simulink library "DAQ_lib_HallPositionTorque"  (R2014b)
settings: Solver=ode45  StartTime=0.0  StopTime=10.0  RelTol=1e-3
undefined symbols (not defined in the file): A_lpf_velocity, ANOMALY_INIT, B1_lpf_velocity, B2_lpf_velocity, Calibration, EnableFT, EncoderAngleLimits, EncoderFiltSys, EncoderThreshold, FTCalibration, GearOffsets, IMUAngleLimits, IMUCommand, IMUThreshold, IMUTorsoOffsets, m_XR17D15x, MAX_ANOMALY, MedullaCommand, MicrostrainFiltSys, MODBUS_TIMEOUT, ResetDAQ, ResetYaw, sample_time, standard, STREAMING_TIMEOUT, TareFT, TorsoCOMOffsets, Ts, TsCAN, TsKVH, UseMicrostrainRate
libraries: xpcethercatlib x207, simulink x53, canmsglib x21, speedgoatlib x13, slrtlib x5, speedgoatlib_IO601 x5, dspswit3 x2, dspmtrx3 x2, xpcseriallib x1, SpeedgoatModified x1
(part 6 of 7)

== system DAQ_lib_HallPositionTorque/DAQ Safety Stops IMU Elmo Amplifiers Position and Torque Control with Hall Sensors/DAQ/EtherCATNetwork/EtherCATRobotMicrostrain/LegElmo_1R/Subsystem1/ShutdownControlWord ==
  Action Port : ActionPort
  Constant : Constant  Value=6  OutDataTypeStr=uint16
  ControlWord : Outport
  wires:
  Constant/1 -> ControlWord/1

== system DAQ_lib_HallPositionTorque/DAQ Safety Stops IMU Elmo Amplifiers Position and Torque Control with Hall Sensors/DAQ/EtherCATNetwork/EtherCATRobotMicrostrain/LegElmo_2L/Subsystem1/EnableControlWord ==
  Action Port : ActionPort
  Constant : Constant  Value=15  OutDataTypeStr=uint16
  ControlWord : Outport
  wires:
  Constant/1 -> ControlWord/1

== system DAQ_lib_HallPositionTorque/DAQ Safety Stops IMU Elmo Amplifiers Position and Torque Control with Hall Sensors/DAQ/EtherCATNetwork/EtherCATRobotMicrostrain/LegElmo_2L/Subsystem1/FaultReset ==
  Action Port : ActionPort
  Constant : Constant  Value=128  OutDataTypeStr=uint16
  ControlWord : Outport
  wires:
  Constant/1 -> ControlWord/1

== system DAQ_lib_HallPositionTorque/DAQ Safety Stops IMU Elmo Amplifiers Position and Torque Control with Hall Sensors/DAQ/EtherCATNetwork/EtherCATRobotMicrostrain/LegElmo_2L/Subsystem1/NothingControlWord ==
  Action Port : ActionPort
  Constant : Constant  Value=0  OutDataTypeStr=uint16
  ControlWord : Outport
  wires:
  Constant/1 -> ControlWord/1

== system DAQ_lib_HallPositionTorque/DAQ Safety Stops IMU Elmo Amplifiers Position and Torque Control with Hall Sensors/DAQ/EtherCATNetwork/EtherCATRobotMicrostrain/LegElmo_2L/Subsystem1/ShutdownControlWord ==
  Action Port : ActionPort
  Constant : Constant  Value=6  OutDataTypeStr=uint16
  ControlWord : Outport
  wires:
  Constant/1 -> ControlWord/1

== system DAQ_lib_HallPositionTorque/DAQ Safety Stops IMU Elmo Amplifiers Position and Torque Control with Hall Sensors/DAQ/EtherCATNetwork/EtherCATRobotMicrostrain/LegElmo_2R/Subsystem1/EnableControlWord ==
  Action Port : ActionPort
  Constant : Constant  Value=15  OutDataTypeStr=uint16
  ControlWord : Outport
  wires:
  Constant/1 -> ControlWord/1

== system DAQ_lib_HallPositionTorque/DAQ Safety Stops IMU Elmo Amplifiers Position and Torque Control with Hall Sensors/DAQ/EtherCATNetwork/EtherCATRobotMicrostrain/LegElmo_2R/Subsystem1/FaultReset ==
  Action Port : ActionPort
  Constant : Constant  Value=128  OutDataTypeStr=uint16
  ControlWord : Outport
  wires:
  Constant/1 -> ControlWord/1

== system DAQ_lib_HallPositionTorque/DAQ Safety Stops IMU Elmo Amplifiers Position and Torque Control with Hall Sensors/DAQ/EtherCATNetwork/EtherCATRobotMicrostrain/LegElmo_2R/Subsystem1/NothingControlWord ==
  Action Port : ActionPort
  Constant : Constant  Value=0  OutDataTypeStr=uint16
  ControlWord : Outport
  wires:
  Constant/1 -> ControlWord/1

== system DAQ_lib_HallPositionTorque/DAQ Safety Stops IMU Elmo Amplifiers Position and Torque Control with Hall Sensors/DAQ/EtherCATNetwork/EtherCATRobotMicrostrain/LegElmo_2R/Subsystem1/ShutdownControlWord ==
  Action Port : ActionPort
  Constant : Constant  Value=6  OutDataTypeStr=uint16
  ControlWord : Outport
  wires:
  Constant/1 -> ControlWord/1

== system DAQ_lib_HallPositionTorque/DAQ Safety Stops IMU Elmo Amplifiers Position and Torque Control with Hall Sensors/DAQ/SerialInterfaces/FTCAN/Read_and_Process_Subsystem/CalibrationMatrixBlock/Fx ==
  In : Inport
  Enable : EnablePort
  Out : Outport
  wires:
  In/1 -> Out/1

== system DAQ_lib_HallPositionTorque/DAQ Safety Stops IMU Elmo Amplifiers Position and Torque Control with Hall Sensors/DAQ/SerialInterfaces/FTCAN/Read_and_Process_Subsystem/CalibrationMatrixBlock/Fy ==
  In : Inport
  Enable : EnablePort
  Out : Outport
  wires:
  In/1 -> Out/1

== system DAQ_lib_HallPositionTorque/DAQ Safety Stops IMU Elmo Amplifiers Position and Torque Control with Hall Sensors/DAQ/SerialInterfaces/FTCAN/Read_and_Process_Subsystem/CalibrationMatrixBlock/Fz ==
  In : Inport
  Enable : EnablePort
  Out : Outport
  wires:
  In/1 -> Out/1

== system DAQ_lib_HallPositionTorque/DAQ Safety Stops IMU Elmo Amplifiers Position and Torque Control with Hall Sensors/DAQ/SerialInterfaces/FTCAN/Read_and_Process_Subsystem/CalibrationMatrixBlock/Tx ==
  In : Inport
  Enable : EnablePort
  Out : Outport
  wires:
  In/1 -> Out/1

== system DAQ_lib_HallPositionTorque/DAQ Safety Stops IMU Elmo Amplifiers Position and Torque Control with Hall Sensors/DAQ/SerialInterfaces/FTCAN/Read_and_Process_Subsystem/CalibrationMatrixBlock/Ty ==
  In : Inport
  Enable : EnablePort
  Out : Outport
  wires:
  In/1 -> Out/1

== system DAQ_lib_HallPositionTorque/DAQ Safety Stops IMU Elmo Amplifiers Position and Torque Control with Hall Sensors/DAQ/SerialInterfaces/FTCAN/Read_and_Process_Subsystem/CalibrationMatrixBlock/Tz ==
  In : Inport
  Enable : EnablePort
  Out : Outport
  wires:
  In/1 -> Out/1

== system DAQ_lib_HallPositionTorque/DAQ Safety Stops IMU Elmo Amplifiers Position and Torque Control with Hall Sensors/DAQ/SerialInterfaces/FTCAN/Read_and_Process_Subsystem/CalibrationMatrixBlock1/Fx ==
  In : Inport
  Enable : EnablePort
  Out : Outport
  wires:
  In/1 -> Out/1

== system DAQ_lib_HallPositionTorque/DAQ Safety Stops IMU Elmo Amplifiers Position and Torque Control with Hall Sensors/DAQ/SerialInterfaces/FTCAN/Read_and_Process_Subsystem/CalibrationMatrixBlock1/Fy ==
  In : Inport
  Enable : EnablePort
  Out : Outport
  wires:
  In/1 -> Out/1

== system DAQ_lib_HallPositionTorque/DAQ Safety Stops IMU Elmo Amplifiers Position and Torque Control with Hall Sensors/DAQ/SerialInterfaces/FTCAN/Read_and_Process_Subsystem/CalibrationMatrixBlock1/Fz ==
  In : Inport
  Enable : EnablePort
  Out : Outport
  wires:
  In/1 -> Out/1

== system DAQ_lib_HallPositionTorque/DAQ Safety Stops IMU Elmo Amplifiers Position and Torque Control with Hall Sensors/DAQ/SerialInterfaces/FTCAN/Read_and_Process_Subsystem/CalibrationMatrixBlock1/Tx ==
  In : Inport
  Enable : EnablePort
  Out : Outport
  wires:
  In/1 -> Out/1

== system DAQ_lib_HallPositionTorque/DAQ Safety Stops IMU Elmo Amplifiers Position and Torque Control with Hall Sensors/DAQ/SerialInterfaces/FTCAN/Read_and_Process_Subsystem/CalibrationMatrixBlock1/Ty ==
  In : Inport
  Enable : EnablePort
  Out : Outport
  wires:
  In/1 -> Out/1

== system DAQ_lib_HallPositionTorque/DAQ Safety Stops IMU Elmo Amplifiers Position and Torque Control with Hall Sensors/DAQ/SerialInterfaces/FTCAN/Read_and_Process_Subsystem/CalibrationMatrixBlock1/Tz ==
  In : Inport
  Enable : EnablePort
  Out : Outport
  wires:
  In/1 -> Out/1

== system DAQ_lib_HallPositionTorque/DAQ Safety Stops IMU Elmo Amplifiers Position and Torque Control with Hall Sensors/DAQ/SerialInterfaces/FTCAN/Read_and_Process_Subsystem/ReadCalibrationMatrixRow_FlipFlops/Subsystem ==
  Status : Inport
  Reset : Inport  Port=2
  Enable : EnablePort
  Logical Operator : Logic  IconShape=distinctive  AllPortsSameDT=off  OutDataTypeStr=boolean
  Logical Operator1 : Logic  Operator=NOT  IconShape=distinctive  AllPortsSameDT=off  OutDataTypeStr=boolean
  StatusLatched : Outport
  wires:
  Status/1 -> Logical Operator/1
  Reset/1 -> Logical Operator1/1
  Logical Operator1/1 -> Logical Operator/2
  Logical Operator/1 -> StatusLatched/1

== system DAQ_lib_HallPositionTorque/DAQ Safety Stops IMU Elmo Amplifiers Position and Torque Control with Hall Sensors/DAQ/SerialInterfaces/FTCAN/Read_and_Process_Subsystem/ReadCalibrationMatrixRow_FlipFlops/Subsystem1 ==
  Status : Inport
  Reset : Inport  Port=2
  Enable : EnablePort
  Logical Operator : Logic  IconShape=distinctive  AllPortsSameDT=off  OutDataTypeStr=boolean
  Logical Operator1 : Logic  Operator=NOT  IconShape=distinctive  AllPortsSameDT=off  OutDataTypeStr=boolean
  StatusLatched : Outport
  wires:
  Status/1 -> Logical Operator/1
  Reset/1 -> Logical Operator1/1
  Logical Operator1/1 -> Logical Operator/2
  Logical Operator/1 -> StatusLatched/1

== system DAQ_lib_HallPositionTorque/DAQ Safety Stops IMU Elmo Amplifiers Position and Torque Control with Hall Sensors/DAQ/SerialInterfaces/FTCAN/Read_and_Process_Subsystem/ReadCalibrationMatrixRow_FlipFlops/Subsystem2 ==
  Status : Inport
  Reset : Inport  Port=2
  Enable : EnablePort
  Logical Operator : Logic  IconShape=distinctive  AllPortsSameDT=off  OutDataTypeStr=boolean
  Logical Operator1 : Logic  Operator=NOT  IconShape=distinctive  AllPortsSameDT=off  OutDataTypeStr=boolean
  StatusLatched : Outport
  wires:
  Status/1 -> Logical Operator/1
  Reset/1 -> Logical Operator1/1
  Logical Operator1/1 -> Logical Operator/2
  Logical Operator/1 -> StatusLatched/1

== system DAQ_lib_HallPositionTorque/DAQ Safety Stops IMU Elmo Amplifiers Position and Torque Control with Hall Sensors/DAQ/SerialInterfaces/FTCAN/Read_and_Process_Subsystem/ReadCalibrationMatrixRow_FlipFlops1/Subsystem ==
  Status : Inport
  Reset : Inport  Port=2
  Enable : EnablePort
  Logical Operator : Logic  IconShape=distinctive  AllPortsSameDT=off  OutDataTypeStr=boolean
  Logical Operator1 : Logic  Operator=NOT  IconShape=distinctive  AllPortsSameDT=off  OutDataTypeStr=boolean
  StatusLatched : Outport
  wires:
  Status/1 -> Logical Operator/1
  Reset/1 -> Logical Operator1/1
  Logical Operator1/1 -> Logical Operator/2
  Logical Operator/1 -> StatusLatched/1

== system DAQ_lib_HallPositionTorque/DAQ Safety Stops IMU Elmo Amplifiers Position and Torque Control with Hall Sensors/DAQ/SerialInterfaces/FTCAN/Read_and_Process_Subsystem/ReadCalibrationMatrixRow_FlipFlops1/Subsystem1 ==
  Status : Inport
  Reset : Inport  Port=2
  Enable : EnablePort
  Logical Operator : Logic  IconShape=distinctive  AllPortsSameDT=off  OutDataTypeStr=boolean
  Logical Operator1 : Logic  Operator=NOT  IconShape=distinctive  AllPortsSameDT=off  OutDataTypeStr=boolean
  StatusLatched : Outport
  wires:
  Status/1 -> Logical Operator/1
  Reset/1 -> Logical Operator1/1
  Logical Operator1/1 -> Logical Operator/2
  Logical Operator/1 -> StatusLatched/1

== system DAQ_lib_HallPositionTorque/DAQ Safety Stops IMU Elmo Amplifiers Position and Torque Control with Hall Sensors/DAQ/SerialInterfaces/FTCAN/Read_and_Process_Subsystem/ReadCalibrationMatrixRow_FlipFlops1/Subsystem2 ==
  Status : Inport
  Reset : Inport  Port=2
  Enable : EnablePort
  Logical Operator : Logic  IconShape=distinctive  AllPortsSameDT=off  OutDataTypeStr=boolean
  Logical Operator1 : Logic  Operator=NOT  IconShape=distinctive  AllPortsSameDT=off  OutDataTypeStr=boolean
  StatusLatched : Outport
  wires:
  Status/1 -> Logical Operator/1
  Reset/1 -> Logical Operator1/1
  Logical Operator1/1 -> Logical Operator/2
  Logical Operator/1 -> StatusLatched/1

== system DAQ_lib_HallPositionTorque/DAQ Safety Stops IMU Elmo Amplifiers Position and Torque Control with Hall Sensors/DAQ/SerialInterfaces/FTCAN/Read_and_Process_Subsystem/Select_SetCalibrationMatrixColumn_From_CommandNo/ReadRow1 ==
  Action Port : ActionPort
  Constant : Constant
  OutValue : Outport
  wires:
  Constant/1 -> OutValue/1

== system DAQ_lib_HallPositionTorque/DAQ Safety Stops IMU Elmo Amplifiers Position and Torque Control with Hall Sensors/DAQ/SerialInterfaces/FTCAN/Read_and_Process_Subsystem/Select_SetCalibrationMatrixColumn_From_CommandNo/ReadRow2 ==
  Action Port : ActionPort
  Constant : Constant  Value=2
  OutValue : Outport
  wires:
  Constant/1 -> OutValue/1

== system DAQ_lib_HallPositionTorque/DAQ Safety Stops IMU Elmo Amplifiers Position and Torque Control with Hall Sensors/DAQ/SerialInterfaces/FTCAN/Read_and_Process_Subsystem/Select_SetCalibrationMatrixColumn_From_CommandNo/ReadRow3 ==
  Action Port : ActionPort
  Constant : Constant  Value=3
  OutValue : Outport
  wires:
  Constant/1 -> OutValue/1

== system DAQ_lib_HallPositionTorque/DAQ Safety Stops IMU Elmo Amplifiers Position and Torque Control with Hall Sensors/DAQ/SerialInterfaces/FTCAN/Read_and_Process_Subsystem/Select_SetCalibrationMatrixColumn_From_CommandNo/ReadRow4 ==
  Action Port : ActionPort
  Constant : Constant  Value=4
  OutValue : Outport
  wires:
  Constant/1 -> OutValue/1

== system DAQ_lib_HallPositionTorque/DAQ Safety Stops IMU Elmo Amplifiers Position and Torque Control with Hall Sensors/DAQ/SerialInterfaces/FTCAN/Read_and_Process_Subsystem/Select_SetCalibrationMatrixColumn_From_CommandNo/ReadRow5 ==
  Action Port : ActionPort
  Constant : Constant  Value=5
  OutValue : Outport
  wires:
  Constant/1 -> OutValue/1

== system DAQ_lib_HallPositionTorque/DAQ Safety Stops IMU Elmo Amplifiers Position and Torque Control with Hall Sensors/DAQ/SerialInterfaces/FTCAN/Read_and_Process_Subsystem/Select_SetCalibrationMatrixColumn_From_CommandNo/ReadRow6 ==
  Action Port : ActionPort
  Constant : Constant  Value=6
  OutValue : Outport
  wires:
  Constant/1 -> OutValue/1

== system DAQ_lib_HallPositionTorque/DAQ Safety Stops IMU Elmo Amplifiers Position and Torque Control with Hall Sensors/DAQ/SerialInterfaces/FTCAN/Read_and_Process_Subsystem/Select_SetCalibrationMatrixColumn_From_CommandNo1/ReadRow1 ==
  Action Port : ActionPort
  Constant : Constant
  OutValue : Outport
  wires:
  Constant/1 -> OutValue/1

== system DAQ_lib_HallPositionTorque/DAQ Safety Stops IMU Elmo Amplifiers Position and Torque Control with Hall Sensors/DAQ/SerialInterfaces/FTCAN/Read_and_Process_Subsystem/Select_SetCalibrationMatrixColumn_From_CommandNo1/ReadRow2 ==
  Action Port : ActionPort
  Constant : Constant  Value=2
  OutValue : Outport
  wires:
  Constant/1 -> OutValue/1

== system DAQ_lib_HallPositionTorque/DAQ Safety Stops IMU Elmo Amplifiers Position and Torque Control with Hall Sensors/DAQ/SerialInterfaces/FTCAN/Read_and_Process_Subsystem/Select_SetCalibrationMatrixColumn_From_CommandNo1/ReadRow3 ==
  Action Port : ActionPort
  Constant : Constant  Value=3
  OutValue : Outport
  wires:
  Constant/1 -> OutValue/1

== system DAQ_lib_HallPositionTorque/DAQ Safety Stops IMU Elmo Amplifiers Position and Torque Control with Hall Sensors/DAQ/SerialInterfaces/FTCAN/Read_and_Process_Subsystem/Select_SetCalibrationMatrixColumn_From_CommandNo1/ReadRow4 ==
  Action Port : ActionPort
  Constant : Constant  Value=4
  OutValue : Outport
  wires:
  Constant/1 -> OutValue/1

== system DAQ_lib_HallPositionTorque/DAQ Safety Stops IMU Elmo Amplifiers Position and Torque Control with Hall Sensors/DAQ/SerialInterfaces/FTCAN/Read_and_Process_Subsystem/Select_SetCalibrationMatrixColumn_From_CommandNo1/ReadRow5 ==
  Action Port : ActionPort
  Constant : Constant  Value=5
  OutValue : Outport
  wires:
  Constant/1 -> OutValue/1

== system DAQ_lib_HallPositionTorque/DAQ Safety Stops IMU Elmo Amplifiers Position and Torque Control with Hall Sensors/DAQ/SerialInterfaces/FTCAN/Read_and_Process_Subsystem/Select_SetCalibrationMatrixColumn_From_CommandNo1/ReadRow6 ==
  Action Port : ActionPort
  Constant : Constant  Value=6
  OutValue : Outport
  wires:
  Constant/1 -> OutValue/1

== system DAQ_lib_HallPositionTorque/DAQ Safety Stops IMU Elmo Amplifiers Position and Torque Control with Hall Sensors/DAQ/SerialInterfaces/FTInterface/Subsystem/ComputeCalibratedTorques/Latch ==
  Gauge : Inport
  Tare : EnablePort
  Bias : Outport  InitialOutput=zeros(6,1,'uint16')
  wires:
  Gauge/1 -> Bias/1

== matlab function DAQ_lib_HallPositionTorque/DAQ Safety Stops IMU Elmo Amplifiers Position and Torque Control with Hall Sensors/AdjustForCOMOffset ==
  data: q_in input; q output; TorsoCOMOffsets input
function q = fcn(q_in, TorsoCOMOffsets)
    %#codegen
    
    TorsoCOMRollOffset  = TorsoCOMOffsets(1)*pi/180;
    TorsoCOMPitchOffset = TorsoCOMOffsets(2)*pi/180;
    
    q = q_in;
    q(2)  = q(2)  + TorsoCOMRollOffset;
    q(10) = q(10) - TorsoCOMRollOffset;
    q(13) = q(13) + TorsoCOMRollOffset;
    
    q(3) = q(3) + TorsoCOMPitchOffset;
    q([4:9 11:12]) = q([4:9 11:12]) - TorsoCOMPitchOffset;
end

== matlab function DAQ_lib_HallPositionTorque/DAQ Safety Stops IMU Elmo Amplifiers Position and Torque Control with Hall Sensors/DAQ/EtherCATNetwork/ComputeEulerAngles ==
  data: RkIn input; wk input; RCal input; Reset input; R0In input; ZYX output; dZYX output; Rk output; R0 output; YawRolloverIn input; YawRollover output
function [ZYX, dZYX, Rk, R0, YawRollover] = fcn(RkIn, wk, RCal, Reset, R0In, YawRolloverIn) %#codegen
    % Convert from IMU frame to robot frame and compute Euler angles. The
    % yaw angle is zeroed whenever (Reset) is true.
        
    if (Reset)
        % Compute the rotation matrix which zeroes the initial yaw
        qT0 = M_to_ZYX(RkIn*RCal);
        R0  = Rz(-qT0(1));
    else
        R0 = R0In;
    end
    
    % Transform from IMU to robot frame and zero initial yaw
    Rk = R0*RkIn*RCal;
    
    % Convert Rk to ZYX Euler angles
    ZYX = M_to_ZYX(Rk);
    
    % Unroll yaw
    YawRolloverCount = YawRolloverIn(1);
    PreviousYaw      = YawRolloverIn(2);
    CurrentYaw       = ZYX(1);
    YawRolloverCount = YawRolloverCount + getYawRollover(CurrentYaw, PreviousYaw);
    YawRollover      = [YawRolloverCount; CurrentYaw];
    ZYX(1)           = ZYX(1) + 2*pi*YawRolloverCount;
    
    % Compute Euler angle derivatives
    qzT = ZYX(1);
    qyT = ZYX(2);
    
    if cos(qyT)>1e-3
        dZYX = [0 -sin(qzT) cos(qzT)*cos(qyT); 0 cos(qzT) sin(qzT)*cos(qyT); 1 0 -sin(qyT)]\(R0*RkIn*wk);
    else
        dZYX = [0; 0; 0];
    end
end

function R = Rz(t)
    R = [cos(t) -sin(t) 0; sin(t) cos(t) 0; 0 0 1];
end

function Rollover = getYawRollover(CurrentYaw, PreviousYaw)
    % Determine if a rollover has occurred on yaw angle If a rollover is
    % detected, the output Rollover is either +1 or -1, depending on the
    % direction of the rollover.
  
    if (PreviousYaw>0 && CurrentYaw < (PreviousYaw-pi))
        Rollover = 1;
    elseif (PreviousYaw<0 && CurrentYaw > (PreviousYaw+pi))
        Rollover = -1;
    else
        Rollover = 0;
    end
end

== stateflow chart DAQ_lib_HallPositionTorque/DAQ Safety Stops IMU Elmo Amplifiers Position and Torque Control with Hall Sensors/DAQ/EtherCATNetwork/EncoderFilters/CheckAndFilterEncoder/AnomalyDetection ==
  state Run
    state Nominal
      en, du:
      q_clean = q;
      q_last = q;
      dq_last = dq;
      Counter_last = Counter;
      ErrorCount = 0;
    state MissedPacket
      en, du:
      q_clean = q_last + dq_last*ANOMALY_DT;
      ErrorCount--;
    state Error
      en: dq_last = dq; //dq is delayed to prevent algebraic loops
      en, du:
      ErrorCount++;
      q_clean = q_last + ErrorCount*dq_last*ANOMALY_DT;
    (default) -> Nominal
    Nominal -> MissedPacket [order 1] : [0 && Counter == Counter_last]
    MissedPacket -> Nominal
    Nominal -> Error [order 2] : [check_error()]
    Error -> Nominal [order 2] : [!check_error()]
  state Init
    en, du:
    q_clean = q;
    q_last = q;
    dq_last = dq;
    ErrorCount = 0;
  (default) -> Init
  Init -> Run : [!Reset && after(ANOMALY_INIT, tick)]
  Run -> Init : [Reset]
  Error -> Init [order 1] : [ErrorCount>MAX_ANOMALY]
  data: err function_output boolean; q input size=1; dq input size=1; Counter input; q_clean output double size=1; ErrorCount output double; MAX_ANOMALY parameter double size=1; q_last local double size=1; dq_last local double size=1; ANOMALY_INIT parameter double size=1; q_limits input double size=2; Threshold input size=1; Reset input boolean size=1; ANOMALY_DT input double size=1; Counter_last local double size=1
  function err = check_error:
    | function err = check_error
    |     %#codegen
    |     err = (q<q_limits(1)) || (q>q_limits(2)) ...
    |         || (abs(q - q_clean) > (ErrorCount+1)*Threshold);
    | end

== matlab function DAQ_lib_HallPositionTorque/DAQ Safety Stops IMU Elmo Amplifiers Position and Torque Control with Hall Sensors/DAQ/EtherCATNetwork/EtherCATRobotMicrostrain/ConvertAmpCurrent ==
  data: adc_value input; measuredCurrent output
function measuredCurrent = convert(adc_value)
    %#codegen

    measuredCurrent = (adc_value) * 60.0 / 8192;
end

== matlab function DAQ_lib_HallPositionTorque/DAQ Safety Stops IMU Elmo Amplifiers Position and Torque Control with Hall Sensors/DAQ/EtherCATNetwork/EtherCATRobotMicrostrain/ConvertLogicVoltage ==
  data: adc_value input; logicVoltage output
function logicVoltage = convert(adc_value)
    %#codegen
    
    MEDULLA_ADC_MAX_VOLTS     = 2.70;
    MEDULLA_ADC_OFFSET_COUNTS = 172;
    
    logicVoltage = (adc_value - MEDULLA_ADC_OFFSET_COUNTS) * (MEDULLA_ADC_MAX_VOLTS/(4095.0))  * 6.0;
end

== matlab function DAQ_lib_HallPositionTorque/DAQ Safety Stops IMU Elmo Amplifiers Position and Torque Control with Hall Sensors/DAQ/EtherCATNetwork/EtherCATRobotMicrostrain/ConvertMotorVoltage ==
  data: adc_value input; motorVoltage output
function motorVoltage = convert(adc_value)
    %#codegen
    
    MOTOR_VOLTAGE_C_OFFSET    = 1300.0;
    MOTOR_VOLTAGE_V_CAL       = 60.2;
    MOTOR_VOLTAGE_C_CAL       = 3600.0;
    
    motorVoltage = (adc_value - MOTOR_VOLTAGE_C_OFFSET)*MOTOR_VOLTAGE_V_CAL/(MOTOR_VOLTAGE_C_CAL-MOTOR_VOLTAGE_C_OFFSET);
end

== matlab function DAQ_lib_HallPositionTorque/DAQ Safety Stops IMU Elmo Amplifiers Position and Torque Control with Hall Sensors/DAQ/EtherCATNetwork/EtherCATRobotMicrostrain/ConvertThermistors ==
  data: Temperatures output; adc_value input
function Temperatures  = convert(adc_value)
    %#codegen
    MEDULLA_ADC_MAX_VOLTS     = 2.70;
    MEDULLA_ADC_OFFSET_COUNTS = 172;
    
    processedADCValue = (adc_value - MEDULLA_ADC_OFFSET_COUNTS) * (MEDULLA_ADC_MAX_VOLTS/(4095.0));
    Temperatures = zeros(30,1); % 20141104
    % Temperatures = (1.0./( (1.0/298.15) + (1.0/3988.0)*log(4700.0./((3.26./processedADCValue) - 1.0)/10000))) - 273.15;
end

== matlab function DAQ_lib_HallPositionTorque/DAQ Safety Stops IMU Elmo Amplifiers Position and Torque Control with Hall Sensors/DAQ/EtherCATNetwork/EtherCATRobotMicrostrain/EncodeSwitches ==
  data: Switches input; LimitSwitchesEncoded output
function LimitSwitchesEncoded = EncodeSwitches(Switches)
    LimitSwitchesVec     = uint32(Switches);
    LimitSwitchesEncoded = double(EncodeSwitches(LimitSwitchesVec));
end

== matlab function DAQ_lib_HallPositionTorque/DAQ Safety Stops IMU Elmo Amplifiers Position and Torque Control with Hall Sensors/DAQ/EtherCATNetwork/EtherCATRobotMicrostrain/IMU_Medulla/TypecastAndCast ==
  data: u input uint32; y output
function y = unit32_to_double(u)
    %#codegen
    ys = typecast(u, 'single');
    y  = double(ys);
end

== matlab function DAQ_lib_HallPositionTorque/DAQ Safety Stops IMU Elmo Amplifiers Position and Torque Control with Hall Sensors/DAQ/EtherCATNetwork/EtherCATRobotMicrostrain/IMU_Medulla/TypecastAndCast1 ==
  data: u input uint32; y output
function y = unit32_to_double(u)
    %#codegen
    ys = typecast(u, 'single');
    y  = double(ys);
end

== matlab function DAQ_lib_HallPositionTorque/DAQ Safety Stops IMU Elmo Amplifiers Position and Torque Control with Hall Sensors/DAQ/EtherCATNetwork/EtherCATRobotMicrostrain/IMU_Medulla/TypecastAndCast2 ==
  data: u input uint32; y output
function y = unit32_to_double(u)
    %#codegen
    ys = typecast(u, 'single');
    y  = double(ys);
end

== stateflow chart DAQ_lib_HallPositionTorque/DAQ Safety Stops IMU Elmo Amplifiers Position and Torque Control with Hall Sensors/DAQ/EtherCATNetwork/EtherCATRobotMicrostrain/LegElmo_1L/State Flow ==
  state Start1
    entry:
    ControlWordIndex = 0;
    Enable = 0;
    FaultDetected = 0;
  note: 2 = Medulla Run
  state Initialization
    state SwitchOnDisabled
      entry:
      ControlWordIndex = 1;
      Timeout = 0;
      Enable = 0;
      FaultDetected = 0;
      during:
      Timeout = Timeout + 1;
    state Fault
      entry:
      ControlWordIndex = 3;
      Enable = 0;
      Timeout = 0;
      FaultDetected = 0;
      during:
      Timeout = Timeout + 1;
      ControlWordIndex = 0;
    state ReadyToSwitchOn
      entry:
      ControlWordIndex = 2;
      Timeout = 0;
      Enable = 0;
      FaultDetected = 0;
      during:
      Timeout = Timeout + 1;
    (default) -> SwitchOnDisabled
    SwitchOnDisabled -> Fault [order 2] : [FaultMode == 1]
    Fault -> Fault [order 1] : [Timeout >=20]
    ReadyToSwitchOn -> SwitchOnDisabled [order 2] : [SwitchOnDisabledMode == 1]
    Fault -> SwitchOnDisabled [order 2] : [SwitchOnDisabledMode == 1]
    SwitchOnDisabled -> ReadyToSwitchOn [order 1] : [ReadyToSwitchOnMode == 1]
    ReadyToSwitchOn -> Fault [order 1] : [FaultMode == 1]
  state FaultRunning
    entry:
    ControlWordIndex = 1;
    Enable = 0;
    FaultDetected = 1;
  note: 5 = Error
  note: 4 = Halt
  state Running
    entry:
    FaultDetected = 0;
    ControlWordIndex = 2;
    Enable = 1;
  (default) -> Start1
  Start1 -> Initialization : [MedullaCommand == 2]
  Initialization -> FaultRunning : [MedullaCommand == 4 || MedullaCommand == 5 ]
  Running -> FaultRunning [order 1] : [FaultMode == 1]
  Running -> FaultRunning [order 2] : [MedullaCommand == 4 || MedullaCommand == 5 ]
  ReadyToSwitchOn -> Running [order 3] : [EnabledMode == 1 && FaultMode == 0]
  data: SwitchOnDisabledMode input; EnabledMode input; ReadyToSwitchOnMode input; ControlWordIndex output; Enable output; Timeout local; FaultMode input; FaultDetected output; MedullaCommand input

== stateflow chart DAQ_lib_HallPositionTorque/DAQ Safety Stops IMU Elmo Amplifiers Position and Torque Control with Hall Sensors/DAQ/EtherCATNetwork/EtherCATRobotMicrostrain/LegElmo_1R/State Flow ==
  state Start1
    entry:
    ControlWordIndex = 0;
    Enable = 0;
    FaultDetected = 0;
  note: 2 = Medulla Run
  state Initialization
    state SwitchOnDisabled
      entry:
      ControlWordIndex = 1;
      Timeout = 0;
      Enable = 0;
      FaultDetected = 0;
      during:
      Timeout = Timeout + 1;
    state Fault
      entry:
      ControlWordIndex = 3;
      Enable = 0;
      Timeout = 0;
      FaultDetected = 0;
      during:
      Timeout = Timeout + 1;
      ControlWordIndex = 0;
    state ReadyToSwitchOn
      entry:
      ControlWordIndex = 2;
      Timeout = 0;
      Enable = 0;
      FaultDetected = 0;
      during:
      Timeout = Timeout + 1;
    (default) -> SwitchOnDisabled
    SwitchOnDisabled -> Fault [order 2] : [FaultMode == 1]
    Fault -> Fault [order 1] : [Timeout >=20]
    ReadyToSwitchOn -> SwitchOnDisabled [order 2] : [SwitchOnDisabledMode == 1]
    Fault -> SwitchOnDisabled [order 2] : [SwitchOnDisabledMode == 1]
    SwitchOnDisabled -> ReadyToSwitchOn [order 1] : [ReadyToSwitchOnMode == 1]
    ReadyToSwitchOn -> Fault [order 1] : [FaultMode == 1]
  state FaultRunning
    entry:
    ControlWordIndex = 1;
    Enable = 0;
    FaultDetected = 1;
  note: 5 = Error
  note: 4 = Halt
  state Running
    entry:
    FaultDetected = 0;
    ControlWordIndex = 2;
    Enable = 1;
  (default) -> Start1
  Start1 -> Initialization : [MedullaCommand == 2]
  Initialization -> FaultRunning : [MedullaCommand == 4 || MedullaCommand == 5 ]
  Running -> FaultRunning [order 1] : [FaultMode == 1]
  Running -> FaultRunning [order 2] : [MedullaCommand == 4 || MedullaCommand == 5 ]
  ReadyToSwitchOn -> Running [order 3] : [EnabledMode == 1 && FaultMode == 0]
  data: SwitchOnDisabledMode input; EnabledMode input; ReadyToSwitchOnMode input; ControlWordIndex output; Enable output; Timeout local; FaultMode input; FaultDetected output; MedullaCommand input

== stateflow chart DAQ_lib_HallPositionTorque/DAQ Safety Stops IMU Elmo Amplifiers Position and Torque Control with Hall Sensors/DAQ/EtherCATNetwork/EtherCATRobotMicrostrain/LegElmo_2L/State Flow ==
  state Start1
    entry:
    ControlWordIndex = 0;
    Enable = 0;
    FaultDetected = 0;
  note: 2 = Medulla Run
  state Initialization
    state SwitchOnDisabled
      entry:
      ControlWordIndex = 1;
      Timeout = 0;
      Enable = 0;
      FaultDetected = 0;
      during:
      Timeout = Timeout + 1;
    state Fault
      entry:
      ControlWordIndex = 3;
      Enable = 0;
      Timeout = 0;
      FaultDetected = 0;
      during:
      Timeout = Timeout + 1;
      ControlWordIndex = 0;
    state ReadyToSwitchOn
      entry:
      ControlWordIndex = 2;
      Timeout = 0;
      Enable = 0;
      FaultDetected = 0;
      during:
      Timeout = Timeout + 1;
    (default) -> SwitchOnDisabled
    SwitchOnDisabled -> Fault [order 2] : [FaultMode == 1]
    Fault -> Fault [order 1] : [Timeout >=20]
    ReadyToSwitchOn -> SwitchOnDisabled [order 2] : [SwitchOnDisabledMode == 1]
    Fault -> SwitchOnDisabled [order 2] : [SwitchOnDisabledMode == 1]
    SwitchOnDisabled -> ReadyToSwitchOn [order 1] : [ReadyToSwitchOnMode == 1]
    ReadyToSwitchOn -> Fault [order 1] : [FaultMode == 1]
  state FaultRunning
    entry:
    ControlWordIndex = 1;
    Enable = 0;
    FaultDetected = 1;
  note: 5 = Error
  note: 4 = Halt
  state Running
    entry:
    FaultDetected = 0;
    ControlWordIndex = 2;
    Enable = 1;
  (default) -> Start1
  Start1 -> Initialization : [MedullaCommand == 2]
  Initialization -> FaultRunning : [MedullaCommand == 4 || MedullaCommand == 5 ]
  Running -> FaultRunning [order 1] : [FaultMode == 1]
  Running -> FaultRunning [order 2] : [MedullaCommand == 4 || MedullaCommand == 5 ]
  ReadyToSwitchOn -> Running [order 3] : [EnabledMode == 1 && FaultMode == 0]
  data: SwitchOnDisabledMode input; EnabledMode input; ReadyToSwitchOnMode input; ControlWordIndex output; Enable output; Timeout local; FaultMode input; FaultDetected output; MedullaCommand input

== stateflow chart DAQ_lib_HallPositionTorque/DAQ Safety Stops IMU Elmo Amplifiers Position and Torque Control with Hall Sensors/DAQ/EtherCATNetwork/EtherCATRobotMicrostrain/LegElmo_2R/State Flow ==
  state Start1
    entry:
    ControlWordIndex = 0;
    Enable = 0;
    FaultDetected = 0;
  note: 2 = Medulla Run
  state Initialization
    state SwitchOnDisabled
      entry:
      ControlWordIndex = 1;
      Timeout = 0;
      Enable = 0;
      FaultDetected = 0;
      during:
      Timeout = Timeout + 1;
    state Fault
      entry:
      ControlWordIndex = 3;
      Enable = 0;
      Timeout = 0;
      FaultDetected = 0;
      during:
      Timeout = Timeout + 1;
      ControlWordIndex = 0;
    state ReadyToSwitchOn
      entry:
      ControlWordIndex = 2;
      Timeout = 0;
      Enable = 0;
      FaultDetected = 0;
      during:
      Timeout = Timeout + 1;
    (default) -> SwitchOnDisabled
    SwitchOnDisabled -> Fault [order 2] : [FaultMode == 1]
    Fault -> Fault [order 1] : [Timeout >=20]
    ReadyToSwitchOn -> SwitchOnDisabled [order 2] : [SwitchOnDisabledMode == 1]
    Fault -> SwitchOnDisabled [order 2] : [SwitchOnDisabledMode == 1]
    SwitchOnDisabled -> ReadyToSwitchOn [order 1] : [ReadyToSwitchOnMode == 1]
    ReadyToSwitchOn -> Fault [order 1] : [FaultMode == 1]
  state FaultRunning
    entry:
    ControlWordIndex = 1;
    Enable = 0;
    FaultDetected = 1;
  note: 5 = Error
  note: 4 = Halt
  state Running
    entry:
    FaultDetected = 0;
    ControlWordIndex = 2;
    Enable = 1;
  (default) -> Start1
  Start1 -> Initialization : [MedullaCommand == 2]
  Initialization -> FaultRunning : [MedullaCommand == 4 || MedullaCommand == 5 ]
  Running -> FaultRunning [order 1] : [FaultMode == 1]
  Running -> FaultRunning [order 2] : [MedullaCommand == 4 || MedullaCommand == 5 ]
  ReadyToSwitchOn -> Running [order 3] : [EnabledMode == 1 && FaultMode == 0]
  data: SwitchOnDisabledMode input; EnabledMode input; ReadyToSwitchOnMode input; ControlWordIndex output; Enable output; Timeout local; FaultMode input; FaultDetected output; MedullaCommand input

== stateflow chart DAQ_lib_HallPositionTorque/DAQ Safety Stops IMU Elmo Amplifiers Position and Torque Control with Hall Sensors/DAQ/EtherCATNetwork/IMUFilters/CheckAndFilterIMU/AnomalyDetection ==
  state Run
    state Nominal
      en, du:
      q_clean = q;
      q_last = q;
      dq_last = dq;
      ErrorCount = 0;
    state Error
      en: dq_last = dq; //dq is delayed to prevent algebraic loops
      en, du:
      ErrorCount++;
      q_clean = q_last + ErrorCount*dq_last*ANOMALY_DT;
    (default) -> Nominal
    Nominal -> Error : [check_error()]
    Error -> Nominal [order 2] : [!check_error()]
  state Init
    en, du:
    q_clean = q;
    q_last = q;
    dq_last = dq;
    ErrorCount = 0;
  (default) -> Init
  Init -> Run : [!Reset && after(ANOMALY_INIT, tick)]
  Run -> Init : [Reset]
  Error -> Init [order 1] : [ErrorCount>MAX_ANOMALY]
  data: err function_output boolean; q input size=1; dq input size=1; q_clean output double size=1; ErrorCount output double; MAX_ANOMALY parameter double size=1; q_last local double size=1; dq_last local double size=1; ANOMALY_INIT parameter double size=1; q_limits input double size=2; Threshold input size=1; Reset input boolean size=1; ANOMALY_DT input double size=1
  function err = check_error:
    | function err = check_error
    |     %#codegen
    |     err = (q<q_limits(1)) || (q>q_limits(2)) || (abs(q - q_clean) > (ErrorCount+1)*Threshold); 
    | end

== matlab function DAQ_lib_HallPositionTorque/DAQ Safety Stops IMU Elmo Amplifiers Position and Torque Control with Hall Sensors/DAQ/EtherCATNetwork/ZeroingLegs ==
  data: u input; u_zeroed output
function u_zeroed = ZeroingLegs(u)

% leg_motor_1R_torque_cmd = u(1);
% leg_motor_2R_torque_cmd = u(2);
% hip_motor_3R_torque_cmd = u(3);
% leg_motor_1L_torque_cmd = u(4);
% leg_motor_2L_torque_cmd = u(5);
% hip_motor_3L_torque_cmd = u(6);

u_zeroed = [0;
            0;
            u(3);
            0;
            0;
            u(6)];

end

== matlab function DAQ_lib_HallPositionTorque/DAQ Safety Stops IMU Elmo Amplifiers Position and Torque Control with Hall Sensors/DAQ/EtherCATNetwork/calibrate ==
  data: Calibration input; AbsEncoders input; IncEncoders input; IncEncodersPrev input; AbsAngle output; Reset input; IncAngle output; RolloverIn input; Rollover output; IncCalTickIn input; IncCalTick output
function [AbsAngle, IncAngle, Rollover, IncCalTick] = calibrate(Calibration,AbsEncoders,IncEncoders,IncEncodersPrev,Reset,RolloverIn,IncCalTickIn)
    %#codegen
    [AbsAngle, IncAngle, Rollover, IncCalTick] = calibrateEncoders2(Calibration,AbsEncoders,IncEncoders,IncEncodersPrev,Reset,RolloverIn,IncCalTickIn);
end

== matlab function DAQ_lib_HallPositionTorque/DAQ Safety Stops IMU Elmo Amplifiers Position and Torque Control with Hall Sensors/DAQ/EtherCATNetwork/convert_mtr_current_to_pwm ==
  data: params input; u input; y output; Reset input
function y = convert_to_pwm(params,u,Reset)
%#codegen
%This function takes motor torque command inputs and outputs
%pwm commands (for the Medulla) in UMich convention

y = zeros(6,1);

if (Reset)
    return
end

%The inputs, which are commanded motor torques 
leg_motor_1R_torque_cmd = u(1);
leg_motor_2R_torque_cmd = u(2);
hip_motor_3R_torque_cmd = u(3);
leg_motor_1L_torque_cmd = u(4);
leg_motor_2L_torque_cmd = u(5);
hip_motor_3L_torque_cmd = u(6);

%Parameters determined experimentally at U Mich
UMich_LEFT_MOTOR_HIP_DIRECTION = params(1); %The direction for the left hip motor. (UMich convention)
UMich_RIGHT_MOTOR_HIP_DIRECTION = params(2); %The direction for the right hip motor. (UMich convention)

% The parameters, from http://code.google.com/p/atrias/source/browse/robot_definitions/
%From robot_invariant_defs.h
MTR_MAX_COUNT = params(3); %The maximum commanded amplifier value. This is the maximum value sent to the Medullas for the amplifier command.
%From biped2_variant_defs.h
MTR_MAX_TORQUE = params(4); %Maximum motor torque for scaling
MTR_HIP_MAX_TORQUE = params(5); %Maximum hip motor torque for scaling
%From leg3_definitions.h (corresponds to our left leg)
%(Note that A=shin and B=thigh for OSU convention)
LEG3_MOTOR_A_DIRECTION = params(6);
LEG3_MOTOR_B_DIRECTION = params(7);
%From leg4_definitions.h (corresponds to our right leg)
%(Note that A=shin and B=thigh for OSU convention)
LEG4_MOTOR_A_DIRECTION = params(8);
LEG4_MOTOR_B_DIRECTION = params(9);

leg_torque_to_pwm = MTR_MAX_COUNT/MTR_MAX_TORQUE;
hip_torque_to_pwm = MTR_MAX_COUNT/MTR_HIP_MAX_TORQUE;

%Convert leg_motor_1L_torque_cmd
leg_motor_1L_direction = LEG3_MOTOR_A_DIRECTION;
y(1) = motor_torque_to_pwm(leg_motor_1L_direction,leg_torque_to_pwm,leg_motor_1L_torque_cmd);

%Convert leg_motor_2L_torque_cmd
leg_motor_2L_direction = LEG3_MOTOR_B_DIRECTION;
y(2) = motor_torque_to_pwm(leg_motor_2L_direction,leg_torque_to_pwm,leg_motor_2L_torque_cmd);

%Convert leg_motor_1R_torque_cmd
leg_motor_1R_direction = LEG4_MOTOR_A_DIRECTION;
y(3) = motor_torque_to_pwm(leg_motor_1R_direction,leg_torque_to_pwm,leg_motor_1R_torque_cmd);

%Convert leg_motor_2R_torque_cmd
leg_motor_2R_direction = LEG4_MOTOR_B_DIRECTION;
y(4) = motor_torque_to_pwm(leg_motor_2R_direction,leg_torque_to_pwm,leg_motor_2R_torque_cmd);

%Convert hip_motor_3R_torque_cmd
hip_motor_3R_direction = UMich_RIGHT_MOTOR_HIP_DIRECTION; %Verified experimentally
y(5) = motor_torque_to_pwm(hip_motor_3R_direction,hip_torque_to_pwm,hip_motor_3R_torque_cmd);

%Convert hip_motor_3L_torque_cmd
hip_motor_3L_direction = UMich_LEFT_MOTOR_HIP_DIRECTION; %Verified experimentally
y(6) = motor_torque_to_pwm(hip_motor_3L_direction,hip_torque_to_pwm,hip_motor_3L_torque_cmd);

end

function motor_pwm = motor_torque_to_pwm(motor_direction,torque_to_pwm_const,motor_torque_cmd)
   motor_pwm = motor_direction*torque_to_pwm_const*motor_torque_cmd;
end

== matlab function DAQ_lib_HallPositionTorque/DAQ Safety Stops IMU Elmo Amplifiers Position and Torque Control with Hall Sensors/DAQ/EtherCATNetwork/qToHall ==
  data: offsets input; hallPositions output; q_in input
function hallPositions  = qToHall(offsets, q_in)
    
    scale = (1/10)*pi/180;
    
    hallPositions = (q_in-offsets)./scale;

end

== stateflow chart DAQ_lib_HallPositionTorque/DAQ Safety Stops IMU Elmo Amplifiers Position and Torque Control with Hall Sensors/DAQ/SerialInterfaces/FTCAN/Chart ==
  state Initialize
    entry:
    SetCommand = 1;
    EnableCommand = 0;
    Timeout = 0;
    NumberOfReadCycles = 1;
    during:
    Timeout = Timeout + 1;
  note: Waste 20 ms
  state SetActiveCalibration
    entry:
    EnableCommand = 1;
    SetCommand = 1;
    Timeout = 0;
    during:
    EnableCommand = 0;
    Timeout = Timeout + 1;
  note: Waits until both devices report being calibrated properly.
      | If not, resend command every 20 ms
  state ResetStoredStatuses5
    entry:
    ResetCalibrationReadFlag = true;
    exit:
    ResetCalibrationReadFlag = false;
  state ResetStoredStatuses4
    entry:
    ResetCalibrationReadFlag = true;
    exit:
    ResetCalibrationReadFlag = false;
  state ResetStoredStatuses3
    entry:
    ResetCalibrationReadFlag = true;
    exit:
    ResetCalibrationReadFlag = false;
  state ResetStoredStatuses
    entry:
    ResetCalibrationReadFlag = true;
    exit:
    ResetCalibrationReadFlag = false;
  state ResetStoredStatuses1
    entry:
    ResetCalibrationReadFlag = true;
    exit:
    ResetCalibrationReadFlag = false;
  state ResetStoredStatuses2
    entry:
    ResetCalibrationReadFlag = true;
    exit:
    ResetCalibrationReadFlag = false;
  state ReadActiveCalibrationMatrix5
    entry:
    EnableCommand = 1;
    SetCommand = 7;
    Timeout = 0;
    during:
    EnableCommand = 0;
    Timeout = Timeout + 1;
  state ReadActiveCalibrationMatrix4
    entry:
    EnableCommand = 1;
    SetCommand = 6;
    Timeout = 0;
    during:
    EnableCommand = 0;
    Timeout = Timeout + 1;
  state ReadActiveCalibrationMatrix3
    entry:
    EnableCommand = 1;
    SetCommand = 5;
    Timeout = 0;
    during:
    EnableCommand = 0;
    Timeout = Timeout + 1;
  state ReadActiveCalibrationMatrix1
    entry:
    EnableCommand = 1;
    SetCommand = 3;
    Timeout = 0;
    during:
    EnableCommand = 0;
    Timeout = Timeout + 1;
  state ReadActiveCalibrationMatrix
    entry:
    EnableCommand = 1;
    SetCommand = 2;
    Timeout = 0;
    during:
    EnableCommand = 0;
    Timeout = Timeout + 1;
  state ReadActiveCalibrationMatrix2
    entry:
    EnableCommand = 1;
    SetCommand = 4;
    Timeout = 0;
    during:
    EnableCommand = 0;
    Timeout = Timeout + 1;
  state ResetStoredStatuses6
    entry:
    ResetCalibrationReadFlag = true;
    exit:
    ResetCalibrationReadFlag = false;
  state StartingStreamMode
    entry:
    NumberOfReadCycles = 4;
    SetCommand = 8;
    EnableCommand = 1;
    Timeout = 0;
    during:
    EnableCommand = 0;
    Timeout = Timeout + 1;
  (default) -> Initialize
  Initialize -> SetActiveCalibration : [Timeout == 20]
  SetActiveCalibration -> SetActiveCalibration [order 2] : [Timeout == 20]
  SetActiveCalibration -> ResetStoredStatuses [order 1] : [SelectedIndex1 == 1 && SelectedIndex2 == 1]
  ReadActiveCalibrationMatrix4 -> ResetStoredStatuses5 [order 2] : [CalibrationRowIsRead1 == 1 && CalibrationRowIsRead2 == 1]
  ReadActiveCalibrationMatrix3 -> ResetStoredStatuses4 [order 2] : [CalibrationRowIsRead1 == 1 && CalibrationRowIsRead2 == 1]
  ReadActiveCalibrationMatrix2 -> ResetStoredStatuses3 [order 2] : [CalibrationRowIsRead1 == 1 && CalibrationRowIsRead2 == 1]
  ReadActiveCalibrationMatrix1 -> ResetStoredStatuses2 [order 2] : [CalibrationRowIsRead1 == 1 && CalibrationRowIsRead2 == 1]
  ResetStoredStatuses5 -> ReadActiveCalibrationMatrix5
  ResetStoredStatuses4 -> ReadActiveCalibrationMatrix4
  ReadActiveCalibrationMatrix -> ResetStoredStatuses1 [order 2] : [CalibrationRowIsRead1 == 1 && CalibrationRowIsRead2 == 1]
  ResetStoredStatuses3 -> ReadActiveCalibrationMatrix3
  ResetStoredStatuses1 -> ReadActiveCalibrationMatrix1
  ResetStoredStatuses2 -> ReadActiveCalibrationMatrix2
  ResetStoredStatuses -> ReadActiveCalibrationMatrix
  ReadActiveCalibrationMatrix5 -> ReadActiveCalibrationMatrix5 [order 1] : [Timeout == 20]
  ReadActiveCalibrationMatrix4 -> ReadActiveCalibrationMatrix4 [order 1] : [Timeout == 20]
  ReadActiveCalibrationMatrix3 -> ReadActiveCalibrationMatrix3 [order 1] : [Timeout == 20]
  ReadActiveCalibrationMatrix1 -> ReadActiveCalibrationMatrix1 [order 1] : [Timeout == 20]
  ReadActiveCalibrationMatrix -> ReadActiveCalibrationMatrix [order 1] : [Timeout == 20]
  ReadActiveCalibrationMatrix2 -> ReadActiveCalibrationMatrix2 [order 1] : [Timeout == 20]
  ReadActiveCalibrationMatrix5 -> ResetStoredStatuses6 [order 2] : [CalibrationRowIsRead1 == 1 && CalibrationRowIsRead2 == 1]
  ResetStoredStatuses6 -> StartingStreamMode
  StartingStreamMode -> StartingStreamMode : [Timeout == 1]
  data: SetCommand output; SelectedIndex1 input; SelectedIndex2 input; EnableCommand output; NumberOfReadCycles output; CalibrationRowIsRead1 input; ResetCalibrationReadFlag output boolean; Timeout output; CalibrationRowIsRead2 input

== matlab function DAQ_lib_HallPositionTorque/DAQ Safety Stops IMU Elmo Amplifiers Position and Torque Control with Hall Sensors/DAQ/SerialInterfaces/FTCAN/ComputeCalibratedTorques/ComputeCalibratedTorques ==
  data: Gauge input; FT output; Bias input; CalibrationMatrix input
function FT = fcn(Gauge, Bias, CalibrationMatrix)
    %#codegen
    FT = CalibrationMatrix * (Gauge - Bias);
    FT(1:3,:) = FT(1:3,:) / 1000; %Cal.CountsPerForce;
    FT(4:6,:) = FT(4:6,:) / 1000; %Cal.CountsPerTorque;
end

== matlab function DAQ_lib_HallPositionTorque/DAQ Safety Stops IMU Elmo Amplifiers Position and Torque Control with Hall Sensors/DAQ/SerialInterfaces/FTCAN/ComputeCalibratedTorques1/ComputeCalibratedTorques ==
  data: Gauge input; FT output; Bias input; CalibrationMatrix input
function FT = fcn(Gauge, Bias, CalibrationMatrix)
    %#codegen
    FT = CalibrationMatrix * (Gauge - Bias);
    FT(1:3,:) = FT(1:3,:) / 1000; %Cal.CountsPerForce;
    FT(4:6,:) = FT(4:6,:) / 1000; %Cal.CountsPerTorque;
end

== matlab function DAQ_lib_HallPositionTorque/DAQ Safety Stops IMU Elmo Amplifiers Position and Torque Control with Hall Sensors/DAQ/SerialInterfaces/FTInterface/Subsystem/ComputeCalibratedTorques/ComputeCalibratedTorques ==
  data: Gauge input; FT output; Bias input; Cal input
function FT = fcn(Gauge, Bias, Cal)
    %#codegen
    FT = Cal.BasicMatrix * (Gauge - Bias);
    FT(1:3,:) = FT(1:3,:) / Cal.CountsPerForce;
    FT(4:6,:) = FT(4:6,:) / Cal.CountsPerTorque;
end
